simulink model "FrancescoGnerreExtraCreditProject"  (R2019b)
settings: Solver=VariableStepAuto  StartTime=0.0  StopTime=10.0  RelTol=1e-3  AbsTol=1e-3
libraries: fl_lib x84, nesl_utility x60, ee_lib x29
settings Model: Creator=franc  LastModifiedBy=franc
settings SolverCC: AutoScaleAbsTol=off
settings DebuggingCC: SymbolicDimsDataTypeCodeGenerationDiagnostic=none
settings SFSimCC: CustomCodeUndefinedFunction=UseInterfaceOnly
settings SimscapeCC: SimscapeLogType=all  SimscapeLogSimulationStatistics=on  SimscapeLogDataHistory=10000

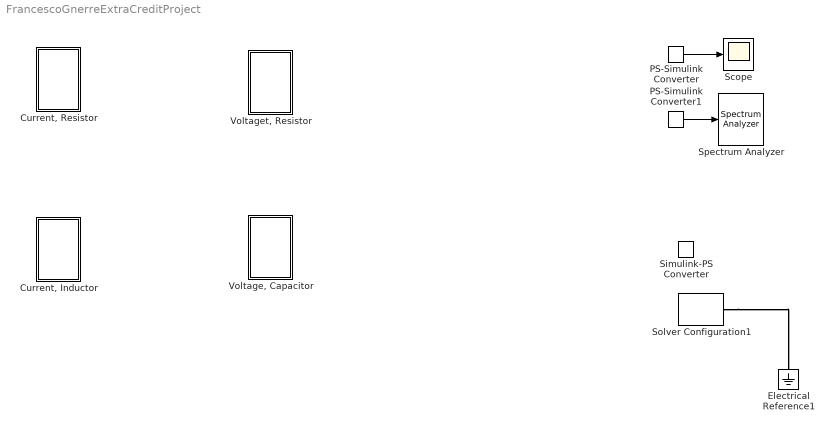
== system FrancescoGnerreExtraCreditProject ==
  "Current, Inductor" : Subsystem
  "Current, Resistor" : Subsystem
  Electrical Reference1 : fl_lib/Electrical/Electrical Elements/Electrical Reference
  PS-Simulink Converter : nesl_utility/PS-Simulink Converter  PhysicalDomain=network_engine_domain  SubClassName=ps_output  LeftPortType=input  RightPortType=output  PseudoPeriodic=off  Frequencies=[]  Unit=inherit  AffineConversion=off
  PS-Simulink Converter1 : nesl_utility/PS-Simulink Converter  PhysicalDomain=network_engine_domain  SubClassName=ps_output  LeftPortType=input  RightPortType=output  PseudoPeriodic=off  Frequencies=[]  Unit=inherit  AffineConversion=off
  Scope : Scope
  Simulink-PS Converter : nesl_utility/Simulink-PS Converter  PhysicalDomain=network_engine_domain  SubClassName=ps_input  LeftPortType=input  RightPortType=output  PseudoPeriodic=off  Frequencies=[]  NoiseDistribution=none  NoiseParameters=[]  Unit=1  AffineConversion=off  FilteringAndDerivatives=provide  SimscapeFilterOrder=1  InputFilterTimeConstant=0.001  UdotUserProvided=0
  Solver Configuration1 : nesl_utility/Solver Configuration  PhysicalDomain=network_engine_domain  SubClassName=solver  LeftPortType=input  RightPortType=generic  Tones=[]  Harmonics=[]  SimulateNoise=off  Profile=off  UseLocalSampling=off  EnableSwitchedLinearOptims=on  FrequencyDomain=off  UseCCode=off  RelTol=0.001  AbsTol=1e-06  MinStep=1e-09  ToWorkspace=off  RevertToSquareIcSolve=off  NumHomotopyIterations=100  PhasorMode=off  PhasorModeNumHarmonics=1  DoDC=off  ResidualTolerance=1e-09  UseLocalSolver=off  LocalSolverChoice=NE_BACKWARD_EULER_ADVANCER  LocalSolverSampleTime=0.001  DoFixedCost=off  MaxNonlinIter=3  MaxModeIter=2  LinearAlgebra=auto  EquationFormulation=NE_TIME_EF  DelaysMemoryBudget=1024  AutomaticFiltering=on  FilteringTimeConstant=0.001  PartitionStorageMethod=AS_NEEDED  PartitionMemoryBudget=1024  PartitionMethod=ROBUST
  Spectrum Analyzer : SpectrumAnalyzer
  "Voltage, Capacitor" : Subsystem
  "Voltaget, Resistor " : Subsystem
  wires:
  PS-Simulink Converter/1 -> Scope/1
  PS-Simulink Converter1/1 -> Spectrum Analyzer/1
  connections:
  Solver Configuration1/RConn1 -- Electrical Reference1/LConn1

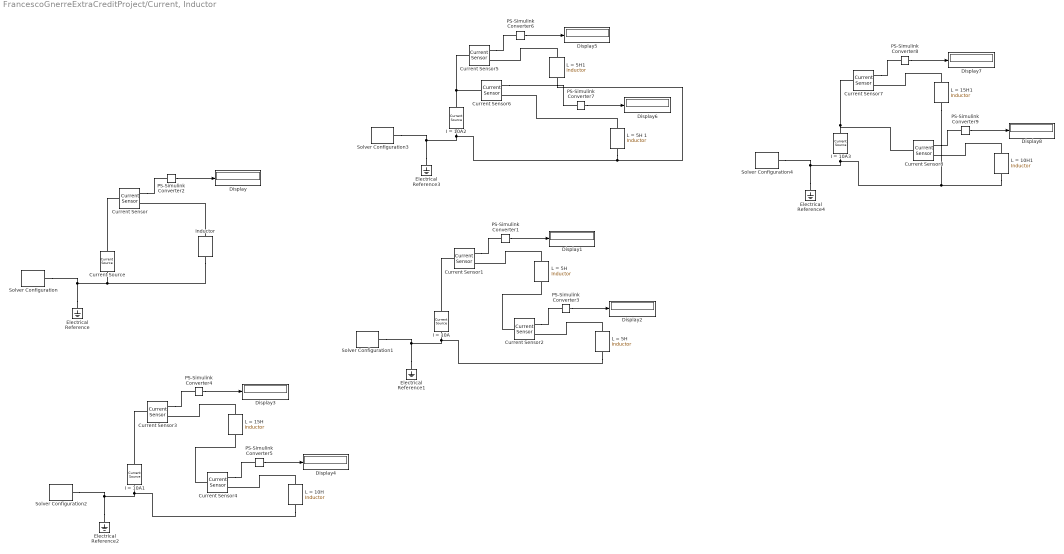
== system FrancescoGnerreExtraCreditProject/Current, Inductor ==
  Current Sensor{,1..8} (9 alike) : fl_lib/Electrical/Electrical Sensors/Current Sensor
  Current Source : ee_lib/Sources/Current Source  dc_current=1 A  ac_current=0 A  ac_shift=0 rad  ac_frequency=60 Hz  noise_mode=0  PSD=0 A^2/Hz  repeatability=1  auto_seed=1578128389  user_seed=0  sample_time=1e-3 s  i_specify=off  i_priority=None  i=0 A  i_nominal_specify=off  i_nominal_unit=A  i_nominal_value=1  v_specify=off  v_priority=None  v=0 V  v_nominal_specify=off  v_nominal_unit=V  v_nominal_value=1
      settings: SourceProductName=Simscape Electrical  SourceProductBaseCode=PS
  Display{,1..8} (9 alike) : Display
  Electrical Reference{,1..4} (5 alike) : fl_lib/Electrical/Electrical Elements/Electrical Reference
  I = 10A : ee_lib/Sources/Current Source  dc_current=10 A  ac_current=0 A  ac_shift=0 rad  ac_frequency=60 Hz  noise_mode=0  PSD=0 A^2/Hz  repeatability=1  auto_seed=1048681922  user_seed=0  sample_time=1e-3 s  i_specify=off  i_priority=None  i=0 A  i_nominal_specify=off  i_nominal_unit=A  i_nominal_value=1  v_specify=off  v_priority=None  v=0 V  v_nominal_specify=off  v_nominal_unit=V  v_nominal_value=1
      settings: SourceProductName=Simscape Electrical  SourceProductBaseCode=PS
  I = 10A1 : ee_lib/Sources/Current Source  dc_current=10 A  ac_current=0 A  ac_shift=0 rad  ac_frequency=60 Hz  noise_mode=0  PSD=0 A^2/Hz  repeatability=1  auto_seed=2238549636  user_seed=0  sample_time=1e-3 s  i_specify=off  i_priority=None  i=0 A  i_nominal_specify=off  i_nominal_unit=A  i_nominal_value=1  v_specify=off  v_priority=None  v=0 V  v_nominal_specify=off  v_nominal_unit=V  v_nominal_value=1
      settings: SourceProductName=Simscape Electrical  SourceProductBaseCode=PS
  I = 10A2 : ee_lib/Sources/Current Source  dc_current=10 A  ac_current=0 A  ac_shift=0 rad  ac_frequency=60 Hz  noise_mode=0  PSD=0 A^2/Hz  repeatability=1  auto_seed=3130446476  user_seed=0  sample_time=1e-3 s  i_specify=off  i_priority=None  i=0 A  i_nominal_specify=off  i_nominal_unit=A  i_nominal_value=1  v_specify=off  v_priority=None  v=0 V  v_nominal_specify=off  v_nominal_unit=V  v_nominal_value=1
      settings: SourceProductName=Simscape Electrical  SourceProductBaseCode=PS
  I = 10A3 : ee_lib/Sources/Current Source  dc_current=10 A  ac_current=0 A  ac_shift=0 rad  ac_frequency=60 Hz  noise_mode=0  PSD=0 A^2/Hz  repeatability=1  auto_seed=2140412339  user_seed=0  sample_time=1e-3 s  i_specify=off  i_priority=None  i=0 A  i_nominal_specify=off  i_nominal_unit=A  i_nominal_value=1  v_specify=off  v_priority=None  v=0 V  v_nominal_specify=off  v_nominal_unit=V  v_nominal_value=1
      settings: SourceProductName=Simscape Electrical  SourceProductBaseCode=PS
  Inductor : ee_lib/Passive/Inductor  l=1e-6 H  L_tol=20  enable_L_tol=0  tol_distribution=1  nSigma=4  r=0 Ohm  g=1e-9 1/Ohm  enable_operating_limits=0  operating_limit_action=2  max_working_current=1 A  power_rating=1 W  enable_faults=0  fault_action=1  lambdaPercent=50  k_faulted=0.9999  turnsShort=0  openCct=0  groundShort=0  groundShortG=0 1/Ohm  tau_fault=1e-3 s  enable_temporal_fault=0  t_fault=1 s  enable_behavioral_fault=0  max_permissible_voltage=100 V  n_fail_on_voltage=1  max_permissible_current=1 A  t_fail_on_current=1 s  i_L_specify=off  i_L_priority=High  i_L=0 A  i_L_nominal_specify=off  i_L_nominal_unit=A  i_L_nominal_value=1
      settings: SourceProductName=Simscape Electrical
  L = 10H : ee_lib/Passive/Inductor  l=10 H  L_tol=20  enable_L_tol=0  tol_distribution=1  nSigma=4  r=0 Ohm  g=1e-9 1/Ohm  enable_operating_limits=0  operating_limit_action=2  max_working_current=1 A  power_rating=1 W  enable_faults=0  fault_action=1  lambdaPercent=50  k_faulted=0.9999  turnsShort=0  openCct=0  groundShort=0  groundShortG=0 1/Ohm  tau_fault=1e-3 s  enable_temporal_fault=0  t_fault=1 s  enable_behavioral_fault=0  max_permissible_voltage=100 V  n_fail_on_voltage=1  max_permissible_current=1 A  t_fail_on_current=1 s  i_L_specify=off  i_L_priority=High  i_L=0 A  i_L_nominal_specify=off  i_L_nominal_unit=A  i_L_nominal_value=1
      settings: SourceProductName=Simscape Electrical
  L = 10H1 : ee_lib/Passive/Inductor  l=10 H  L_tol=20  enable_L_tol=0  tol_distribution=1  nSigma=4  r=0 Ohm  g=1e-9 1/Ohm  enable_operating_limits=0  operating_limit_action=2  max_working_current=1 A  power_rating=1 W  enable_faults=0  fault_action=1  lambdaPercent=50  k_faulted=0.9999  turnsShort=0  openCct=0  groundShort=0  groundShortG=0 1/Ohm  tau_fault=1e-3 s  enable_temporal_fault=0  t_fault=1 s  enable_behavioral_fault=0  max_permissible_voltage=100 V  n_fail_on_voltage=1  max_permissible_current=1 A  t_fail_on_current=1 s  i_L_specify=off  i_L_priority=High  i_L=0 A  i_L_nominal_specify=off  i_L_nominal_unit=A  i_L_nominal_value=1
      settings: SourceProductName=Simscape Electrical
  L = 15H : ee_lib/Passive/Inductor  l=15 H  L_tol=20  enable_L_tol=0  tol_distribution=1  nSigma=4  r=0 Ohm  g=1e-9 1/Ohm  enable_operating_limits=0  operating_limit_action=2  max_working_current=1 A  power_rating=1 W  enable_faults=0  fault_action=1  lambdaPercent=50  k_faulted=0.9999  turnsShort=0  openCct=0  groundShort=0  groundShortG=0 1/Ohm  tau_fault=1e-3 s  enable_temporal_fault=0  t_fault=1 s  enable_behavioral_fault=0  max_permissible_voltage=100 V  n_fail_on_voltage=1  max_permissible_current=1 A  t_fail_on_current=1 s  i_L_specify=off  i_L_priority=High  i_L=0 A  i_L_nominal_specify=off  i_L_nominal_unit=A  i_L_nominal_value=1
      settings: SourceProductName=Simscape Electrical
  L = 15H1 : ee_lib/Passive/Inductor  l=15 H  L_tol=20  enable_L_tol=0  tol_distribution=1  nSigma=4  r=0 Ohm  g=1e-9 1/Ohm  enable_operating_limits=0  operating_limit_action=2  max_working_current=1 A  power_rating=1 W  enable_faults=0  fault_action=1  lambdaPercent=50  k_faulted=0.9999  turnsShort=0  openCct=0  groundShort=0  groundShortG=0 1/Ohm  tau_fault=1e-3 s  enable_temporal_fault=0  t_fault=1 s  enable_behavioral_fault=0  max_permissible_voltage=100 V  n_fail_on_voltage=1  max_permissible_current=1 A  t_fail_on_current=1 s  i_L_specify=off  i_L_priority=High  i_L=0 A  i_L_nominal_specify=off  i_L_nominal_unit=A  i_L_nominal_value=1
      settings: SourceProductName=Simscape Electrical
  L = 5H : ee_lib/Passive/Inductor  l=5 H  L_tol=20  enable_L_tol=0  tol_distribution=1  nSigma=4  r=0 Ohm  g=1e-9 1/Ohm  enable_operating_limits=0  operating_limit_action=2  max_working_current=1 A  power_rating=1 W  enable_faults=0  fault_action=1  lambdaPercent=50  k_faulted=0.9999  turnsShort=0  openCct=0  groundShort=0  groundShortG=0 1/Ohm  tau_fault=1e-3 s  enable_temporal_fault=0  t_fault=1 s  enable_behavioral_fault=0  max_permissible_voltage=100 V  n_fail_on_voltage=1  max_permissible_current=1 A  t_fail_on_current=1 s  i_L_specify=off  i_L_priority=High  i_L=0 A  i_L_nominal_specify=off  i_L_nominal_unit=A  i_L_nominal_value=1
      settings: SourceProductName=Simscape Electrical
  "L = 5H " : ee_lib/Passive/Inductor  l=5 H  L_tol=20  enable_L_tol=0  tol_distribution=1  nSigma=4  r=0 Ohm  g=1e-9 1/Ohm  enable_operating_limits=0  operating_limit_action=2  max_working_current=1 A  power_rating=1 W  enable_faults=0  fault_action=1  lambdaPercent=50  k_faulted=0.9999  turnsShort=0  openCct=0  groundShort=0  groundShortG=0 1/Ohm  tau_fault=1e-3 s  enable_temporal_fault=0  t_fault=1 s  enable_behavioral_fault=0  max_permissible_voltage=100 V  n_fail_on_voltage=1  max_permissible_current=1 A  t_fail_on_current=1 s  i_L_specify=off  i_L_priority=High  i_L=0 A  i_L_nominal_specify=off  i_L_nominal_unit=A  i_L_nominal_value=1
      settings: SourceProductName=Simscape Electrical
  L = 5H 1 : ee_lib/Passive/Inductor  l=5 H  L_tol=20  enable_L_tol=0  tol_distribution=1  nSigma=4  r=0 Ohm  g=1e-9 1/Ohm  enable_operating_limits=0  operating_limit_action=2  max_working_current=1 A  power_rating=1 W  enable_faults=0  fault_action=1  lambdaPercent=50  k_faulted=0.9999  turnsShort=0  openCct=0  groundShort=0  groundShortG=0 1/Ohm  tau_fault=1e-3 s  enable_temporal_fault=0  t_fault=1 s  enable_behavioral_fault=0  max_permissible_voltage=100 V  n_fail_on_voltage=1  max_permissible_current=1 A  t_fail_on_current=1 s  i_L_specify=off  i_L_priority=High  i_L=0 A  i_L_nominal_specify=off  i_L_nominal_unit=A  i_L_nominal_value=1
      settings: SourceProductName=Simscape Electrical
  L = 5H1 : ee_lib/Passive/Inductor  l=5 H  L_tol=20  enable_L_tol=0  tol_distribution=1  nSigma=4  r=0 Ohm  g=1e-9 1/Ohm  enable_operating_limits=0  operating_limit_action=2  max_working_current=1 A  power_rating=1 W  enable_faults=0  fault_action=1  lambdaPercent=50  k_faulted=0.9999  turnsShort=0  openCct=0  groundShort=0  groundShortG=0 1/Ohm  tau_fault=1e-3 s  enable_temporal_fault=0  t_fault=1 s  enable_behavioral_fault=0  max_permissible_voltage=100 V  n_fail_on_voltage=1  max_permissible_current=1 A  t_fail_on_current=1 s  i_L_specify=off  i_L_priority=High  i_L=0 A  i_L_nominal_specify=off  i_L_nominal_unit=A  i_L_nominal_value=1
      settings: SourceProductName=Simscape Electrical
  PS-Simulink Converter{1..9} (9 alike) : nesl_utility/PS-Simulink Converter  PhysicalDomain=network_engine_domain  SubClassName=ps_output  LeftPortType=input  RightPortType=output  PseudoPeriodic=off  Frequencies=[]  Unit=inherit  AffineConversion=off
  Solver Configuration{,1..4} (5 alike) : nesl_utility/Solver Configuration  PhysicalDomain=network_engine_domain  SubClassName=solver  LeftPortType=input  RightPortType=generic  Tones=[]  Harmonics=[]  SimulateNoise=off  Profile=off  UseLocalSampling=off  EnableSwitchedLinearOptims=on  FrequencyDomain=off  UseCCode=off  RelTol=0.001  AbsTol=1e-06  MinStep=1e-09  ToWorkspace=off  RevertToSquareIcSolve=off  NumHomotopyIterations=100  PhasorMode=off  PhasorModeNumHarmonics=1  DoDC=off  ResidualTolerance=1e-09  UseLocalSolver=off  LocalSolverChoice=NE_BACKWARD_EULER_ADVANCER  LocalSolverSampleTime=0.001  DoFixedCost=off  MaxNonlinIter=3  MaxModeIter=2  LinearAlgebra=auto  EquationFormulation=NE_TIME_EF  DelaysMemoryBudget=1024  AutomaticFiltering=on  FilteringTimeConstant=0.001  PartitionStorageMethod=AS_NEEDED  PartitionMemoryBudget=1024  PartitionMethod=ROBUST
  wires:
  PS-Simulink Converter2/1 -> Display/1
  PS-Simulink Converter1/1 -> Display1/1
  PS-Simulink Converter3/1 -> Display2/1
  PS-Simulink Converter4/1 -> Display3/1
  PS-Simulink Converter5/1 -> Display4/1
  PS-Simulink Converter6/1 -> Display5/1
  PS-Simulink Converter7/1 -> Display6/1
  PS-Simulink Converter9/1 -> Display8/1
  PS-Simulink Converter8/1 -> Display7/1
  connections:
  Current Sensor/RConn1 -- PS-Simulink Converter2/LConn1
  Electrical Reference/LConn1 -- Solver Configuration/RConn1 -- Inductor/RConn1 -- Current Source/RConn1
  Inductor/LConn1 -- Current Sensor/RConn2
  Current Source/LConn1 -- Current Sensor/LConn1
  Electrical Reference1/LConn1 -- Solver Configuration1/RConn1 -- "L = 5H "/RConn1 -- I = 10A/RConn1
  I = 10A/LConn1 -- Current Sensor1/LConn1
  Current Sensor1/RConn1 -- PS-Simulink Converter1/LConn1
  L = 5H/LConn1 -- Current Sensor1/RConn2
  "L = 5H "/LConn1 -- Current Sensor2/RConn2
  Current Sensor2/RConn1 -- PS-Simulink Converter3/LConn1
  Current Sensor2/LConn1 -- L = 5H/RConn1
  Electrical Reference2/LConn1 -- Solver Configuration2/RConn1 -- L = 10H/RConn1 -- I = 10A1/RConn1
  L = 15H/LConn1 -- Current Sensor3/RConn2
  Current Sensor4/LConn1 -- L = 15H/RConn1
  Current Sensor3/RConn1 -- PS-Simulink Converter4/LConn1
  Current Sensor4/RConn1 -- PS-Simulink Converter5/LConn1
  L = 10H/LConn1 -- Current Sensor4/RConn2
  I = 10A1/LConn1 -- Current Sensor3/LConn1
  Electrical Reference3/LConn1 -- Solver Configuration3/RConn1 -- L = 5H1/RConn1 -- L = 5H 1/RConn1 -- I = 10A2/RConn1
  L = 5H1/LConn1 -- Current Sensor5/RConn2
  I = 10A2/LConn1 -- Current Sensor6/LConn1 -- Current Sensor5/LConn1
  Current Sensor5/RConn1 -- PS-Simulink Converter6/LConn1
  Current Sensor6/RConn1 -- PS-Simulink Converter7/LConn1
  L = 5H 1/LConn1 -- Current Sensor6/RConn2
  Electrical Reference4/LConn1 -- Solver Configuration4/RConn1 -- L = 10H1/RConn1 -- L = 15H1/RConn1 -- I = 10A3/RConn1
  I = 10A3/LConn1 -- Current Sensor7/LConn1 -- Current Sensor8/LConn1
  L = 10H1/LConn1 -- Current Sensor8/RConn2
  L = 15H1/LConn1 -- Current Sensor7/RConn2
  Current Sensor8/RConn1 -- PS-Simulink Converter9/LConn1
  Current Sensor7/RConn1 -- PS-Simulink Converter8/LConn1

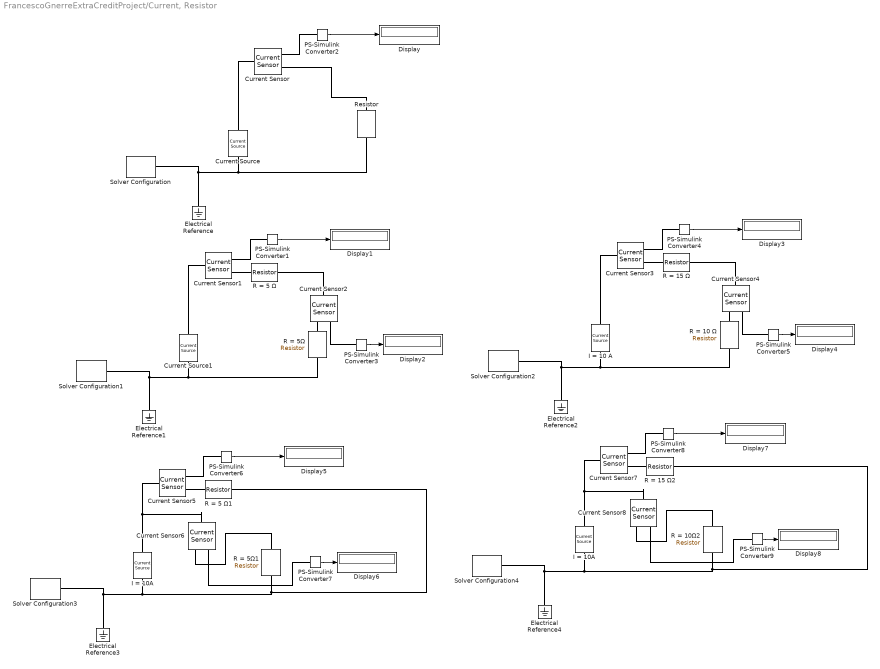
== system FrancescoGnerreExtraCreditProject/Current, Resistor ==
  Current Sensor{,1..8} (9 alike) : fl_lib/Electrical/Electrical Sensors/Current Sensor
  Current Source : ee_lib/Sources/Current Source  dc_current=1 A  ac_current=0 A  ac_shift=0 rad  ac_frequency=60 Hz  noise_mode=0  PSD=0 A^2/Hz  repeatability=1  auto_seed=3346497771  user_seed=0  sample_time=1e-3 s  i_specify=off  i_priority=None  i=0 A  i_nominal_specify=off  i_nominal_unit=A  i_nominal_value=1  v_specify=off  v_priority=None  v=0 V  v_nominal_specify=off  v_nominal_unit=V  v_nominal_value=1
      settings: SourceProductName=Simscape Electrical  SourceProductBaseCode=PS
  Current Source1 : ee_lib/Sources/Current Source  dc_current=10 A  ac_current=0 A  ac_shift=0 rad  ac_frequency=60 Hz  noise_mode=0  PSD=0 A^2/Hz  repeatability=1  auto_seed=2301248012  user_seed=0  sample_time=1e-3 s  i_specify=off  i_priority=None  i=0 A  i_nominal_specify=off  i_nominal_unit=A  i_nominal_value=1  v_specify=off  v_priority=None  v=0 V  v_nominal_specify=off  v_nominal_unit=V  v_nominal_value=1
      settings: SourceProductName=Simscape Electrical  SourceProductBaseCode=PS
  Display{,1..8} (9 alike) : Display
  Electrical Reference{,1..4} (5 alike) : fl_lib/Electrical/Electrical Elements/Electrical Reference
  I = 10 A : ee_lib/Sources/Current Source  dc_current=10 A  ac_current=0 A  ac_shift=0 rad  ac_frequency=60 Hz  noise_mode=0  PSD=0 A^2/Hz  repeatability=1  auto_seed=702280276  user_seed=0  sample_time=1e-3 s  i_specify=off  i_priority=None  i=0 A  i_nominal_specify=off  i_nominal_unit=A  i_nominal_value=1  v_specify=off  v_priority=None  v=0 V  v_nominal_specify=off  v_nominal_unit=V  v_nominal_value=1
      settings: SourceProductName=Simscape Electrical  SourceProductBaseCode=PS
  I = 10A : ee_lib/Sources/Current Source  dc_current=10 A  ac_current=0 A  ac_shift=0 rad  ac_frequency=60 Hz  noise_mode=0  PSD=0 A^2/Hz  repeatability=1  auto_seed=3391863913  user_seed=0  sample_time=1e-3 s  i_specify=off  i_priority=None  i=0 A  i_nominal_specify=off  i_nominal_unit=A  i_nominal_value=1  v_specify=off  v_priority=None  v=0 V  v_nominal_specify=off  v_nominal_unit=V  v_nominal_value=1
      settings: SourceProductName=Simscape Electrical  SourceProductBaseCode=PS
  "I = 10A  " : ee_lib/Sources/Current Source  dc_current=10 A  ac_current=0 A  ac_shift=0 rad  ac_frequency=60 Hz  noise_mode=0  PSD=0 A^2/Hz  repeatability=1  auto_seed=1010892594  user_seed=0  sample_time=1e-3 s  i_specify=off  i_priority=None  i=0 A  i_nominal_specify=off  i_nominal_unit=A  i_nominal_value=1  v_specify=off  v_priority=None  v=0 V  v_nominal_specify=off  v_nominal_unit=V  v_nominal_value=1
      settings: SourceProductName=Simscape Electrical  SourceProductBaseCode=PS
  PS-Simulink Converter{1..9} (9 alike) : nesl_utility/PS-Simulink Converter  PhysicalDomain=network_engine_domain  SubClassName=ps_output  LeftPortType=input  RightPortType=output  PseudoPeriodic=off  Frequencies=[]  Unit=inherit  AffineConversion=off
  R = 10 Ω : fl_lib/Electrical/Electrical Elements/Resistor  R=10 Ohm  i_specify=off  i_priority=None  i=0 A  i_nominal_specify=off  i_nominal_unit=A  i_nominal_value=1  v_specify=off  v_priority=None  v=0 V  v_nominal_specify=off  v_nominal_unit=V  v_nominal_value=1
  R = 10Ω2 : fl_lib/Electrical/Electrical Elements/Resistor  R=10 Ohm  i_specify=off  i_priority=None  i=0 A  i_nominal_specify=off  i_nominal_unit=A  i_nominal_value=1  v_specify=off  v_priority=None  v=0 V  v_nominal_specify=off  v_nominal_unit=V  v_nominal_value=1
  R = 15 Ω : fl_lib/Electrical/Electrical Elements/Resistor  R=15 Ohm  i_specify=off  i_priority=None  i=0 A  i_nominal_specify=off  i_nominal_unit=A  i_nominal_value=1  v_specify=off  v_priority=None  v=0 V  v_nominal_specify=off  v_nominal_unit=V  v_nominal_value=1
  R = 15 Ω2 : fl_lib/Electrical/Electrical Elements/Resistor  R=15 Ohm  i_specify=off  i_priority=None  i=0 A  i_nominal_specify=off  i_nominal_unit=A  i_nominal_value=1  v_specify=off  v_priority=None  v=0 V  v_nominal_specify=off  v_nominal_unit=V  v_nominal_value=1
  R = 5 Ω : fl_lib/Electrical/Electrical Elements/Resistor  R=5 Ohm  i_specify=off  i_priority=None  i=0 A  i_nominal_specify=off  i_nominal_unit=A  i_nominal_value=1  v_specify=off  v_priority=None  v=0 V  v_nominal_specify=off  v_nominal_unit=V  v_nominal_value=1
  R = 5 Ω1 : fl_lib/Electrical/Electrical Elements/Resistor  R=5 Ohm  i_specify=off  i_priority=None  i=0 A  i_nominal_specify=off  i_nominal_unit=A  i_nominal_value=1  v_specify=off  v_priority=None  v=0 V  v_nominal_specify=off  v_nominal_unit=V  v_nominal_value=1
  R = 5Ω : fl_lib/Electrical/Electrical Elements/Resistor  R=5 Ohm  i_specify=off  i_priority=None  i=0 A  i_nominal_specify=off  i_nominal_unit=A  i_nominal_value=1  v_specify=off  v_priority=None  v=0 V  v_nominal_specify=off  v_nominal_unit=V  v_nominal_value=1
  R = 5Ω1 : fl_lib/Electrical/Electrical Elements/Resistor  R=5 Ohm  i_specify=off  i_priority=None  i=0 A  i_nominal_specify=off  i_nominal_unit=A  i_nominal_value=1  v_specify=off  v_priority=None  v=0 V  v_nominal_specify=off  v_nominal_unit=V  v_nominal_value=1
  Resistor : fl_lib/Electrical/Electrical Elements/Resistor  R=1 Ohm  i_specify=off  i_priority=None  i=0 A  i_nominal_specify=off  i_nominal_unit=A  i_nominal_value=1  v_specify=off  v_priority=None  v=0 V  v_nominal_specify=off  v_nominal_unit=V  v_nominal_value=1
  Solver Configuration{,1..4} (5 alike) : nesl_utility/Solver Configuration  PhysicalDomain=network_engine_domain  SubClassName=solver  LeftPortType=input  RightPortType=generic  Tones=[]  Harmonics=[]  SimulateNoise=off  Profile=off  UseLocalSampling=off  EnableSwitchedLinearOptims=on  FrequencyDomain=off  UseCCode=off  RelTol=0.001  AbsTol=1e-06  MinStep=1e-09  ToWorkspace=off  RevertToSquareIcSolve=off  NumHomotopyIterations=100  PhasorMode=off  PhasorModeNumHarmonics=1  DoDC=off  ResidualTolerance=1e-09  UseLocalSolver=off  LocalSolverChoice=NE_BACKWARD_EULER_ADVANCER  LocalSolverSampleTime=0.001  DoFixedCost=off  MaxNonlinIter=3  MaxModeIter=2  LinearAlgebra=auto  EquationFormulation=NE_TIME_EF  DelaysMemoryBudget=1024  AutomaticFiltering=on  FilteringTimeConstant=0.001  PartitionStorageMethod=AS_NEEDED  PartitionMemoryBudget=1024  PartitionMethod=ROBUST
  wires:
  PS-Simulink Converter2/1 -> Display/1
  PS-Simulink Converter1/1 -> Display1/1
  PS-Simulink Converter3/1 -> Display2/1
  PS-Simulink Converter5/1 -> Display4/1
  PS-Simulink Converter4/1 -> Display3/1
  PS-Simulink Converter7/1 -> Display6/1
  PS-Simulink Converter6/1 -> Display5/1
  PS-Simulink Converter9/1 -> Display8/1
  PS-Simulink Converter8/1 -> Display7/1
  connections:
  Current Sensor/RConn2 -- Resistor/LConn1
  Current Sensor/RConn1 -- PS-Simulink Converter2/LConn1
  Solver Configuration/RConn1 -- Resistor/RConn1 -- Current Source/RConn1 -- Electrical Reference/LConn1
  Current Source/LConn1 -- Current Sensor/LConn1
  Electrical Reference1/LConn1 -- Solver Configuration1/RConn1 -- R = 5Ω/RConn1 -- Current Source1/RConn1
  Current Source1/LConn1 -- Current Sensor1/LConn1
  Current Sensor1/RConn1 -- PS-Simulink Converter1/LConn1
  Current Sensor2/RConn1 -- PS-Simulink Converter3/LConn1
  R = 5 Ω/LConn1 -- Current Sensor1/RConn2
  R = 5 Ω/RConn1 -- Current Sensor2/LConn1
  Current Sensor2/RConn2 -- R = 5Ω/LConn1
  Electrical Reference2/LConn1 -- Solver Configuration2/RConn1 -- R = 10 Ω/RConn1 -- I = 10 A/RConn1
  Current Sensor3/RConn1 -- PS-Simulink Converter4/LConn1
  Current Sensor4/RConn1 -- PS-Simulink Converter5/LConn1
  R = 15 Ω/RConn1 -- Current Sensor4/LConn1
  I = 10 A/LConn1 -- Current Sensor3/LConn1
  R = 15 Ω/LConn1 -- Current Sensor3/RConn2
  Current Sensor4/RConn2 -- R = 10 Ω/LConn1
  Electrical Reference3/LConn1 -- Solver Configuration3/RConn1 -- R = 5 Ω1/RConn1 -- R = 5Ω1/RConn1 -- I = 10A/RConn1
  Current Sensor5/RConn1 -- PS-Simulink Converter6/LConn1
  I = 10A/LConn1 -- Current Sensor6/LConn1 -- Current Sensor5/LConn1
  R = 5 Ω1/LConn1 -- Current Sensor5/RConn2
  Current Sensor6/RConn1 -- PS-Simulink Converter7/LConn1
  Current Sensor6/RConn2 -- R = 5Ω1/LConn1
  R = 10Ω2/RConn1 -- R = 15 Ω2/RConn1 -- "I = 10A  "/RConn1 -- Solver Configuration4/RConn1 -- Electrical Reference4/LConn1
  "I = 10A  "/LConn1 -- Current Sensor8/LConn1 -- Current Sensor7/LConn1
  Current Sensor7/RConn1 -- PS-Simulink Converter8/LConn1
  R = 15 Ω2/LConn1 -- Current Sensor7/RConn2
  Current Sensor8/RConn1 -- PS-Simulink Converter9/LConn1
  Current Sensor8/RConn2 -- R = 10Ω2/LConn1

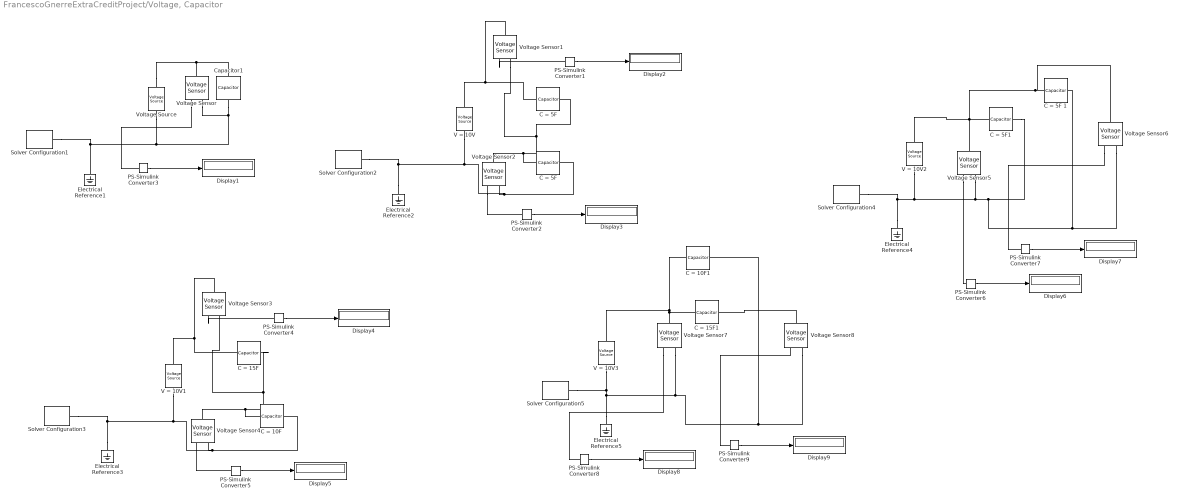
== system FrancescoGnerreExtraCreditProject/Voltage, Capacitor ==
  C = 10F : fl_lib/Electrical/Electrical Elements/Capacitor  c=10 F  r=1e-6 Ohm  g=0 1/Ohm  i_specify=off  i_priority=None  i=0 A  i_nominal_specify=off  i_nominal_unit=A  i_nominal_value=1  v_specify=off  v_priority=None  v=0 V  v_nominal_specify=off  v_nominal_unit=V  v_nominal_value=1  vc_specify=off  vc_priority=High  vc=0 V  vc_nominal_specify=off  vc_nominal_unit=V  vc_nominal_value=1
  C = 10F1 : fl_lib/Electrical/Electrical Elements/Capacitor  c=10 F  r=1e-6 Ohm  g=0 1/Ohm  i_specify=off  i_priority=None  i=0 A  i_nominal_specify=off  i_nominal_unit=A  i_nominal_value=1  v_specify=off  v_priority=None  v=0 V  v_nominal_specify=off  v_nominal_unit=V  v_nominal_value=1  vc_specify=off  vc_priority=High  vc=0 V  vc_nominal_specify=off  vc_nominal_unit=V  vc_nominal_value=1
  C = 15F : fl_lib/Electrical/Electrical Elements/Capacitor  c=15 F  r=1e-6 Ohm  g=0 1/Ohm  i_specify=off  i_priority=None  i=0 A  i_nominal_specify=off  i_nominal_unit=A  i_nominal_value=1  v_specify=off  v_priority=None  v=0 V  v_nominal_specify=off  v_nominal_unit=V  v_nominal_value=1  vc_specify=off  vc_priority=High  vc=0 V  vc_nominal_specify=off  vc_nominal_unit=V  vc_nominal_value=1
  C = 15F1 : fl_lib/Electrical/Electrical Elements/Capacitor  c=15 F  r=1e-6 Ohm  g=0 1/Ohm  i_specify=off  i_priority=None  i=0 A  i_nominal_specify=off  i_nominal_unit=A  i_nominal_value=1  v_specify=off  v_priority=None  v=0 V  v_nominal_specify=off  v_nominal_unit=V  v_nominal_value=1  vc_specify=off  vc_priority=High  vc=0 V  vc_nominal_specify=off  vc_nominal_unit=V  vc_nominal_value=1
  C = 5F : fl_lib/Electrical/Electrical Elements/Capacitor  c=5 F  r=1e-6 Ohm  g=0 1/Ohm  i_specify=off  i_priority=None  i=0 A  i_nominal_specify=off  i_nominal_unit=A  i_nominal_value=1  v_specify=off  v_priority=None  v=0 V  v_nominal_specify=off  v_nominal_unit=V  v_nominal_value=1  vc_specify=off  vc_priority=High  vc=0 V  vc_nominal_specify=off  vc_nominal_unit=V  vc_nominal_value=1
  "C = 5F " : fl_lib/Electrical/Electrical Elements/Capacitor  c=5 F  r=1e-6 Ohm  g=0 1/Ohm  i_specify=off  i_priority=None  i=0 A  i_nominal_specify=off  i_nominal_unit=A  i_nominal_value=1  v_specify=off  v_priority=None  v=0 V  v_nominal_specify=off  v_nominal_unit=V  v_nominal_value=1  vc_specify=off  vc_priority=High  vc=0 V  vc_nominal_specify=off  vc_nominal_unit=V  vc_nominal_value=1
  C = 5F 1 : fl_lib/Electrical/Electrical Elements/Capacitor  c=5 F  r=1e-6 Ohm  g=0 1/Ohm  i_specify=off  i_priority=None  i=0 A  i_nominal_specify=off  i_nominal_unit=A  i_nominal_value=1  v_specify=off  v_priority=None  v=0 V  v_nominal_specify=off  v_nominal_unit=V  v_nominal_value=1  vc_specify=off  vc_priority=High  vc=0 V  vc_nominal_specify=off  vc_nominal_unit=V  vc_nominal_value=1
  C = 5F1 : fl_lib/Electrical/Electrical Elements/Capacitor  c=5 F  r=1e-6 Ohm  g=0 1/Ohm  i_specify=off  i_priority=None  i=0 A  i_nominal_specify=off  i_nominal_unit=A  i_nominal_value=1  v_specify=off  v_priority=None  v=0 V  v_nominal_specify=off  v_nominal_unit=V  v_nominal_value=1  vc_specify=off  vc_priority=High  vc=0 V  vc_nominal_specify=off  vc_nominal_unit=V  vc_nominal_value=1
  Capacitor1 : fl_lib/Electrical/Electrical Elements/Capacitor  c=1e-6 F  r=1e-6 Ohm  g=0 1/Ohm  i_specify=off  i_priority=None  i=0 A  i_nominal_specify=off  i_nominal_unit=A  i_nominal_value=1  v_specify=off  v_priority=None  v=0 V  v_nominal_specify=off  v_nominal_unit=V  v_nominal_value=1  vc_specify=off  vc_priority=High  vc=0 V  vc_nominal_specify=off  vc_nominal_unit=V  vc_nominal_value=1
  Display{1..9} (9 alike) : Display
  Electrical Reference{1..5} (5 alike) : fl_lib/Electrical/Electrical Elements/Electrical Reference
  PS-Simulink Converter{1..9} (9 alike) : nesl_utility/PS-Simulink Converter  PhysicalDomain=network_engine_domain  SubClassName=ps_output  LeftPortType=input  RightPortType=output  PseudoPeriodic=off  Frequencies=[]  Unit=inherit  AffineConversion=off
  Solver Configuration{1..5} (5 alike) : nesl_utility/Solver Configuration  PhysicalDomain=network_engine_domain  SubClassName=solver  LeftPortType=input  RightPortType=generic  Tones=[]  Harmonics=[]  SimulateNoise=off  Profile=off  UseLocalSampling=off  EnableSwitchedLinearOptims=on  FrequencyDomain=off  UseCCode=off  RelTol=0.001  AbsTol=1e-06  MinStep=1e-09  ToWorkspace=off  RevertToSquareIcSolve=off  NumHomotopyIterations=100  PhasorMode=off  PhasorModeNumHarmonics=1  DoDC=off  ResidualTolerance=1e-09  UseLocalSolver=off  LocalSolverChoice=NE_BACKWARD_EULER_ADVANCER  LocalSolverSampleTime=0.001  DoFixedCost=off  MaxNonlinIter=3  MaxModeIter=2  LinearAlgebra=auto  EquationFormulation=NE_TIME_EF  DelaysMemoryBudget=1024  AutomaticFiltering=on  FilteringTimeConstant=0.001  PartitionStorageMethod=AS_NEEDED  PartitionMemoryBudget=1024  PartitionMethod=ROBUST
  V = 10V : ee_lib/Sources/Voltage Source  dc_voltage=10 V  ac_voltage=0 V  ac_shift=0 rad  ac_frequency=60 Hz  noise_mode=0  PSD=0 V^2/Hz  repeatability=1  auto_seed=84271841  user_seed=0  sample_time=1e-3 s  i_specify=off  i_priority=None  i=0 A  i_nominal_specify=off  i_nominal_unit=A  i_nominal_value=1  v_specify=off  v_priority=None  v=0 V  v_nominal_specify=off  v_nominal_unit=V  v_nominal_value=1
      settings: SourceProductName=Simscape Electrical
  V = 10V1 : ee_lib/Sources/Voltage Source  dc_voltage=10 V  ac_voltage=0 V  ac_shift=0 rad  ac_frequency=60 Hz  noise_mode=0  PSD=0 V^2/Hz  repeatability=1  auto_seed=1869064737  user_seed=0  sample_time=1e-3 s  i_specify=off  i_priority=None  i=0 A  i_nominal_specify=off  i_nominal_unit=A  i_nominal_value=1  v_specify=off  v_priority=None  v=0 V  v_nominal_specify=off  v_nominal_unit=V  v_nominal_value=1
      settings: SourceProductName=Simscape Electrical
  V = 10V2 : ee_lib/Sources/Voltage Source  dc_voltage=10 V  ac_voltage=0 V  ac_shift=0 rad  ac_frequency=60 Hz  noise_mode=0  PSD=0 V^2/Hz  repeatability=1  auto_seed=3474586740  user_seed=0  sample_time=1e-3 s  i_specify=off  i_priority=None  i=0 A  i_nominal_specify=off  i_nominal_unit=A  i_nominal_value=1  v_specify=off  v_priority=None  v=0 V  v_nominal_specify=off  v_nominal_unit=V  v_nominal_value=1
      settings: SourceProductName=Simscape Electrical
  V = 10V3 : ee_lib/Sources/Voltage Source  dc_voltage=10 V  ac_voltage=0 V  ac_shift=0 rad  ac_frequency=60 Hz  noise_mode=0  PSD=0 V^2/Hz  repeatability=1  auto_seed=314578156  user_seed=0  sample_time=1e-3 s  i_specify=off  i_priority=None  i=0 A  i_nominal_specify=off  i_nominal_unit=A  i_nominal_value=1  v_specify=off  v_priority=None  v=0 V  v_nominal_specify=off  v_nominal_unit=V  v_nominal_value=1
      settings: SourceProductName=Simscape Electrical
  Voltage Sensor{,1..8} (9 alike) : fl_lib/Electrical/Electrical Sensors/Voltage Sensor
  Voltage Source : ee_lib/Sources/Voltage Source  dc_voltage=1 V  ac_voltage=0 V  ac_shift=0 rad  ac_frequency=60 Hz  noise_mode=0  PSD=0 V^2/Hz  repeatability=1  auto_seed=471147023  user_seed=0  sample_time=1e-3 s  i_specify=off  i_priority=None  i=0 A  i_nominal_specify=off  i_nominal_unit=A  i_nominal_value=1  v_specify=off  v_priority=None  v=0 V  v_nominal_specify=off  v_nominal_unit=V  v_nominal_value=1
      settings: SourceProductName=Simscape Electrical
  wires:
  PS-Simulink Converter3/1 -> Display1/1
  PS-Simulink Converter1/1 -> Display2/1
  PS-Simulink Converter2/1 -> Display3/1
  PS-Simulink Converter5/1 -> Display5/1
  PS-Simulink Converter4/1 -> Display4/1
  PS-Simulink Converter7/1 -> Display7/1
  PS-Simulink Converter6/1 -> Display6/1
  PS-Simulink Converter9/1 -> Display9/1
  PS-Simulink Converter8/1 -> Display8/1
  connections:
  Voltage Sensor/RConn2 -- Capacitor1/RConn1 -- Solver Configuration1/RConn1 -- Electrical Reference1/LConn1 -- Voltage Source/RConn1
  Voltage Source/LConn1 -- Capacitor1/LConn1 -- Voltage Sensor/LConn1
  Voltage Sensor/RConn1 -- PS-Simulink Converter3/LConn1
  Voltage Sensor1/LConn1 -- C = 5F/LConn1 -- V = 10V/LConn1
  C = 10F/LConn1 -- Voltage Sensor4/LConn1 -- C = 15F/RConn1 -- Voltage Sensor3/RConn2
  Voltage Sensor3/LConn1 -- C = 15F/LConn1 -- V = 10V1/LConn1
  Voltage Sensor1/RConn2 -- "C = 5F "/LConn1 -- Voltage Sensor2/LConn1 -- C = 5F/RConn1
  Electrical Reference2/LConn1 -- "C = 5F "/RConn1 -- Voltage Sensor2/RConn2 -- V = 10V/RConn1 -- Solver Configuration2/RConn1
  Electrical Reference3/LConn1 -- C = 10F/RConn1 -- Voltage Sensor4/RConn2 -- V = 10V1/RConn1 -- Solver Configuration3/RConn1
  Voltage Sensor1/RConn1 -- PS-Simulink Converter1/LConn1
  Voltage Sensor3/RConn1 -- PS-Simulink Converter4/LConn1
  Voltage Sensor2/RConn1 -- PS-Simulink Converter2/LConn1
  Voltage Sensor4/RConn1 -- PS-Simulink Converter5/LConn1
  Voltage Sensor5/LConn1 -- Voltage Sensor6/LConn1 -- C = 5F 1/LConn1 -- V = 10V2/LConn1 -- C = 5F1/LConn1
  Electrical Reference4/LConn1 -- Solver Configuration4/RConn1 -- C = 5F1/RConn1 -- Voltage Sensor6/RConn2 -- C = 5F 1/RConn1 -- Voltage Sensor5/RConn2 -- V = 10V2/RConn1
  Voltage Sensor6/RConn1 -- PS-Simulink Converter7/LConn1
  Voltage Sensor5/RConn1 -- PS-Simulink Converter6/LConn1
  Voltage Sensor7/LConn1 -- C = 10F1/LConn1 -- V = 10V3/LConn1 -- C = 15F1/LConn1
  Voltage Sensor8/LConn1 -- C = 15F1/RConn1
  Electrical Reference5/LConn1 -- Voltage Sensor8/RConn2 -- C = 10F1/RConn1 -- Voltage Sensor7/RConn2 -- V = 10V3/RConn1 -- Solver Configuration5/RConn1
  Voltage Sensor7/RConn1 -- PS-Simulink Converter8/LConn1
  Voltage Sensor8/RConn1 -- PS-Simulink Converter9/LConn1

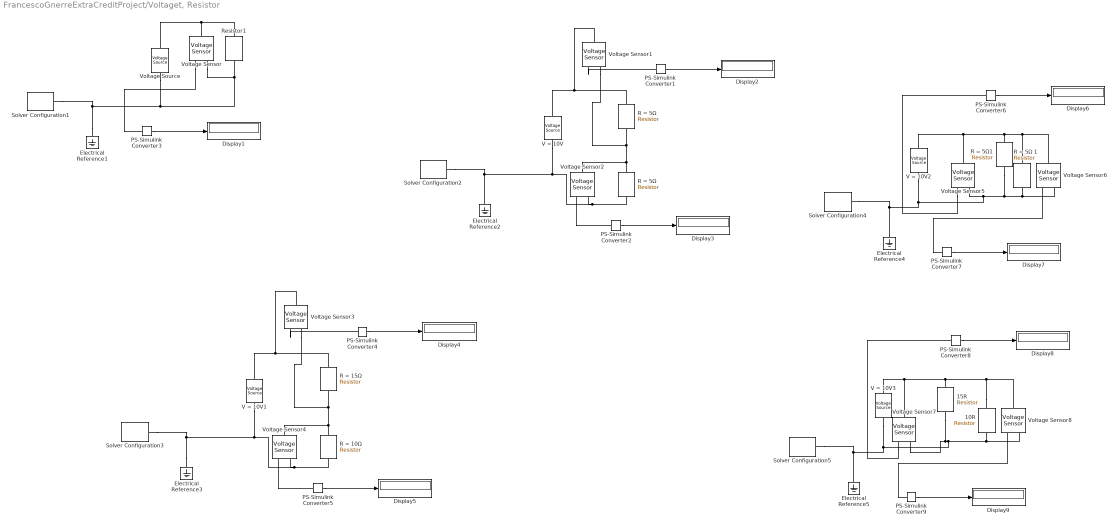
== system FrancescoGnerreExtraCreditProject/Voltaget, Resistor  ==
  10R : fl_lib/Electrical/Electrical Elements/Resistor  R=10 Ohm  i_specify=off  i_priority=None  i=0 A  i_nominal_specify=off  i_nominal_unit=A  i_nominal_value=1  v_specify=off  v_priority=None  v=0 V  v_nominal_specify=off  v_nominal_unit=V  v_nominal_value=1
  15R : fl_lib/Electrical/Electrical Elements/Resistor  R=15 Ohm  i_specify=off  i_priority=None  i=0 A  i_nominal_specify=off  i_nominal_unit=A  i_nominal_value=1  v_specify=off  v_priority=None  v=0 V  v_nominal_specify=off  v_nominal_unit=V  v_nominal_value=1
  Display{1..9} (9 alike) : Display
  Electrical Reference{1..5} (5 alike) : fl_lib/Electrical/Electrical Elements/Electrical Reference
  PS-Simulink Converter{1..9} (9 alike) : nesl_utility/PS-Simulink Converter  PhysicalDomain=network_engine_domain  SubClassName=ps_output  LeftPortType=input  RightPortType=output  PseudoPeriodic=off  Frequencies=[]  Unit=inherit  AffineConversion=off
  R = 10Ω : fl_lib/Electrical/Electrical Elements/Resistor  R=10 Ohm  i_specify=off  i_priority=None  i=0 A  i_nominal_specify=off  i_nominal_unit=A  i_nominal_value=1  v_specify=off  v_priority=None  v=0 V  v_nominal_specify=off  v_nominal_unit=V  v_nominal_value=1
  R = 15Ω : fl_lib/Electrical/Electrical Elements/Resistor  R=15 Ohm  i_specify=off  i_priority=None  i=0 A  i_nominal_specify=off  i_nominal_unit=A  i_nominal_value=1  v_specify=off  v_priority=None  v=0 V  v_nominal_specify=off  v_nominal_unit=V  v_nominal_value=1
  R = 5Ω : fl_lib/Electrical/Electrical Elements/Resistor  R=5 Ohm  i_specify=off  i_priority=None  i=0 A  i_nominal_specify=off  i_nominal_unit=A  i_nominal_value=1  v_specify=off  v_priority=None  v=0 V  v_nominal_specify=off  v_nominal_unit=V  v_nominal_value=1
  "R = 5Ω " : fl_lib/Electrical/Electrical Elements/Resistor  R=5 Ohm  i_specify=off  i_priority=None  i=0 A  i_nominal_specify=off  i_nominal_unit=A  i_nominal_value=1  v_specify=off  v_priority=None  v=0 V  v_nominal_specify=off  v_nominal_unit=V  v_nominal_value=1
  R = 5Ω 1 : fl_lib/Electrical/Electrical Elements/Resistor  R=5 Ohm  i_specify=off  i_priority=None  i=0 A  i_nominal_specify=off  i_nominal_unit=A  i_nominal_value=1  v_specify=off  v_priority=None  v=0 V  v_nominal_specify=off  v_nominal_unit=V  v_nominal_value=1
  R = 5Ω1 : fl_lib/Electrical/Electrical Elements/Resistor  R=5 Ohm  i_specify=off  i_priority=None  i=0 A  i_nominal_specify=off  i_nominal_unit=A  i_nominal_value=1  v_specify=off  v_priority=None  v=0 V  v_nominal_specify=off  v_nominal_unit=V  v_nominal_value=1
  Resistor1 : fl_lib/Electrical/Electrical Elements/Resistor  R=1 Ohm  i_specify=off  i_priority=None  i=0 A  i_nominal_specify=off  i_nominal_unit=A  i_nominal_value=1  v_specify=off  v_priority=None  v=0 V  v_nominal_specify=off  v_nominal_unit=V  v_nominal_value=1
  Solver Configuration{1..5} (5 alike) : nesl_utility/Solver Configuration  PhysicalDomain=network_engine_domain  SubClassName=solver  LeftPortType=input  RightPortType=generic  Tones=[]  Harmonics=[]  SimulateNoise=off  Profile=off  UseLocalSampling=off  EnableSwitchedLinearOptims=on  FrequencyDomain=off  UseCCode=off  RelTol=0.001  AbsTol=1e-06  MinStep=1e-09  ToWorkspace=off  RevertToSquareIcSolve=off  NumHomotopyIterations=100  PhasorMode=off  PhasorModeNumHarmonics=1  DoDC=off  ResidualTolerance=1e-09  UseLocalSolver=off  LocalSolverChoice=NE_BACKWARD_EULER_ADVANCER  LocalSolverSampleTime=0.001  DoFixedCost=off  MaxNonlinIter=3  MaxModeIter=2  LinearAlgebra=auto  EquationFormulation=NE_TIME_EF  DelaysMemoryBudget=1024  AutomaticFiltering=on  FilteringTimeConstant=0.001  PartitionStorageMethod=AS_NEEDED  PartitionMemoryBudget=1024  PartitionMethod=ROBUST
  V = 10V : ee_lib/Sources/Voltage Source  dc_voltage=10 V  ac_voltage=0 V  ac_shift=0 rad  ac_frequency=60 Hz  noise_mode=0  PSD=0 V^2/Hz  repeatability=1  auto_seed=255135218  user_seed=0  sample_time=1e-3 s  i_specify=off  i_priority=None  i=0 A  i_nominal_specify=off  i_nominal_unit=A  i_nominal_value=1  v_specify=off  v_priority=None  v=0 V  v_nominal_specify=off  v_nominal_unit=V  v_nominal_value=1
      settings: SourceProductName=Simscape Electrical
  V = 10V1 : ee_lib/Sources/Voltage Source  dc_voltage=10 V  ac_voltage=0 V  ac_shift=0 rad  ac_frequency=60 Hz  noise_mode=0  PSD=0 V^2/Hz  repeatability=1  auto_seed=3492292942  user_seed=0  sample_time=1e-3 s  i_specify=off  i_priority=None  i=0 A  i_nominal_specify=off  i_nominal_unit=A  i_nominal_value=1  v_specify=off  v_priority=None  v=0 V  v_nominal_specify=off  v_nominal_unit=V  v_nominal_value=1
      settings: SourceProductName=Simscape Electrical
  V = 10V2 : ee_lib/Sources/Voltage Source  dc_voltage=10 V  ac_voltage=0 V  ac_shift=0 rad  ac_frequency=60 Hz  noise_mode=0  PSD=0 V^2/Hz  repeatability=1  auto_seed=3555082614  user_seed=0  sample_time=1e-3 s  i_specify=off  i_priority=None  i=0 A  i_nominal_specify=off  i_nominal_unit=A  i_nominal_value=1  v_specify=off  v_priority=None  v=0 V  v_nominal_specify=off  v_nominal_unit=V  v_nominal_value=1
      settings: SourceProductName=Simscape Electrical
  V = 10V3 : ee_lib/Sources/Voltage Source  dc_voltage=10 V  ac_voltage=0 V  ac_shift=0 rad  ac_frequency=60 Hz  noise_mode=0  PSD=0 V^2/Hz  repeatability=1  auto_seed=820280517  user_seed=0  sample_time=1e-3 s  i_specify=off  i_priority=None  i=0 A  i_nominal_specify=off  i_nominal_unit=A  i_nominal_value=1  v_specify=off  v_priority=None  v=0 V  v_nominal_specify=off  v_nominal_unit=V  v_nominal_value=1
      settings: SourceProductName=Simscape Electrical
  Voltage Sensor{,1..8} (9 alike) : fl_lib/Electrical/Electrical Sensors/Voltage Sensor
  Voltage Source : ee_lib/Sources/Voltage Source  dc_voltage=1 V  ac_voltage=0 V  ac_shift=0 rad  ac_frequency=60 Hz  noise_mode=0  PSD=0 V^2/Hz  repeatability=1  auto_seed=3287869569  user_seed=0  sample_time=1e-3 s  i_specify=off  i_priority=None  i=0 A  i_nominal_specify=off  i_nominal_unit=A  i_nominal_value=1  v_specify=off  v_priority=None  v=0 V  v_nominal_specify=off  v_nominal_unit=V  v_nominal_value=1
      settings: SourceProductName=Simscape Electrical
  wires:
  PS-Simulink Converter3/1 -> Display1/1
  PS-Simulink Converter1/1 -> Display2/1
  PS-Simulink Converter2/1 -> Display3/1
  PS-Simulink Converter4/1 -> Display4/1
  PS-Simulink Converter5/1 -> Display5/1
  PS-Simulink Converter6/1 -> Display6/1
  PS-Simulink Converter7/1 -> Display7/1
  PS-Simulink Converter9/1 -> Display9/1
  PS-Simulink Converter8/1 -> Display8/1
  connections:
  Electrical Reference1/LConn1 -- Voltage Source/RConn1 -- Voltage Sensor/RConn2 -- Resistor1/RConn1 -- Solver Configuration1/RConn1
  Resistor1/LConn1 -- Voltage Sensor/LConn1 -- Voltage Source/LConn1
  Voltage Sensor/RConn1 -- PS-Simulink Converter3/LConn1
  Voltage Sensor1/LConn1 -- V = 10V/LConn1 -- R = 5Ω/LConn1
  Voltage Sensor2/RConn2 -- V = 10V/RConn1 -- Solver Configuration2/RConn1 -- Electrical Reference2/LConn1 -- "R = 5Ω "/RConn1
  Voltage Sensor1/RConn1 -- PS-Simulink Converter1/LConn1
  Voltage Sensor1/RConn2 -- Voltage Sensor2/LConn1 -- "R = 5Ω "/LConn1 -- R = 5Ω/RConn1
  Voltage Sensor2/RConn1 -- PS-Simulink Converter2/LConn1
  Voltage Sensor3/RConn2 -- Voltage Sensor4/LConn1 -- R = 10Ω/LConn1 -- R = 15Ω/RConn1
  Voltage Sensor3/LConn1 -- V = 10V1/LConn1 -- R = 15Ω/LConn1
  Electrical Reference3/LConn1 -- R = 10Ω/RConn1 -- Voltage Sensor4/RConn2 -- V = 10V1/RConn1 -- Solver Configuration3/RConn1
  Voltage Sensor4/RConn1 -- PS-Simulink Converter5/LConn1
  Voltage Sensor3/RConn1 -- PS-Simulink Converter4/LConn1
  Voltage Sensor6/RConn1 -- PS-Simulink Converter7/LConn1
  Voltage Sensor5/RConn1 -- PS-Simulink Converter6/LConn1
  V = 10V2/RConn1 -- R = 5Ω1/RConn1 -- Voltage Sensor6/RConn2 -- R = 5Ω 1/RConn1 -- Voltage Sensor5/RConn2 -- Solver Configuration4/RConn1 -- Electrical Reference4/LConn1
  V = 10V2/LConn1 -- R = 5Ω1/LConn1 -- Voltage Sensor6/LConn1 -- R = 5Ω 1/LConn1 -- Voltage Sensor5/LConn1
  V = 10V3/RConn1 -- Voltage Sensor8/RConn2 -- 10R/RConn1 -- 15R/RConn1 -- Voltage Sensor7/RConn2 -- Solver Configuration5/RConn1 -- Electrical Reference5/LConn1
  10R/LConn1 -- Voltage Sensor7/LConn1 -- V = 10V3/LConn1 -- 15R/LConn1 -- Voltage Sensor8/LConn1
  Voltage Sensor8/RConn1 -- PS-Simulink Converter9/LConn1
  Voltage Sensor7/RConn1 -- PS-Simulink Converter8/LConn1
